simulink library "DT_Library"  (R2025b)
settings: Solver=VariableStepAuto  StartTime=0.0  StopTime=10.0  RelTol=1e-3
undefined symbols (not defined in the file or in its folder): Ala, Arg, Asn, Asp, BMedia, BRX, Choline, CMP, Glc, Glu, Gly, GMP, GSmode, His, Ile, K_ht, K_lt, Lac, Leu, Lys, mAb, Met, Phe, Pro, Ser, Thr, Trp, Tyr, V1, Val, Xv
libraries: simulink x23, $bdroot x15
(part 2 of 2)

== matlab function DT_Library/Vessel/Vessel ==
  settings: updateMethod=DISCRETE
  data: Vesselcondition input Bus: Vessel size=1; dvoldt output size=1; Instream input Bus: Stream size=1; Outflow input size=1; SecondOutflow input size=1; gsrate input size=1; dConcdt output size=31; dAAdt input Bus: AA; AAflux output Bus: AA; Params input; GSmode input
function [dvoldt, dConcdt,AAflux] = vessel(Vesselcondition, Instream, Outflow, SecondOutflow, gsrate,dAAdt, Params, GSmode)
arguments
    Vesselcondition
    Instream
    Outflow 
    SecondOutflow  
    gsrate 
    dAAdt 
    Params 
    GSmode
end
dvoldt = 0;
dConcdt = zeros(31,1);

[dvoldt, dConcdt,AAflux] = DT_VesselCalc(Vesselcondition, Instream, Outflow, Params, SecondOutflow, gsrate,dAAdt,GSmode);

end

== matlab function DT_Library/Stream Join/MATLAB Function ==
  data: A input Bus: Stream; joinedstream output Bus: Stream; B input Bus: Stream
function joinedstream  = fcn(A,B)
    joinedstream = DT_streamjoin(A,B);
end

== matlab function DT_Library/Stream Split/MATLAB Function ==
  data: u input Bus: Stream; Permeate output Bus: Stream; Flowthrough output Bus: Stream; f input
function [Permeate, Flowthrough] = fcn(u,f)

[Permeate, Flowthrough] = DT_splitstream(u,f);

== matlab function DT_Library/DT Cell Retention/CellRet ==
  data: Stream input Bus: Stream; Harv_Stream output Bus: Stream; HarvFlow input; RetEff input; Ret_Stream output Bus: Stream
function [Harv_Stream,Ret_Stream] = CellRet(Stream, HarvFlow, RetEff)
[Harv_Stream, Ret_Stream]=DT_cellretention(Stream, HarvFlow, RetEff);

== matlab function DT_Library/Vessel/GSM/GS model ==
  settings: updateMethod=DISCRETE  sampleTime=1
  data: gsrate output double size=1; AAflux input Bus: AA; onlinereading input Bus: conc; phase input; GSmode input
function gsrate  = gsmodel(AAflux,onlinereading,phase,GSmode)
coder.extrinsic('DT_gsmodel');
    gsrate = 0;
   if GSmode == 1
        if onlinereading.Xv>0
         gsrate = DT_gsmodel(AAflux,phase, GSmode);
        end
   end
end
